simulink model "model"  (R2019a)
settings: Solver=VariableStepAuto  StartTime=0.0  StopTime=Tf  RelTol=5e-3
values from neighbouring files (symbols this model uses):
  d = 0.01    [RUN_model.m]    (also in testing.m; training.m)
  f = 10    [RUN_model.m]    (also in testing.m; training.m)
  J = 0.01    [RUN_model.m]    (also in testing.m; training.m)
  Kb = 0.0301    [RUN_model.m]    (also in testing.m; training.m)
  Kt = 0.03    [RUN_model.m]    (also in testing.m; training.m)
  L = 20e-2    (= 0.2)    [RUN_model.m]    (also in testing.m; training.m)
  La = 0.94e-3    (= 0.00094)    [RUN_model.m]    (also in testing.m; training.m)
  M = 1000e-3    (= 1)    [RUN_model.m]    (also in testing.m; training.m)
  mode = 1    [testing.m]    (also in training.m)
  N = 10    [RUN_model.m]    (also in testing.m; training.m)
  R = 0.02    [RUN_model.m]    (also in testing.m; training.m)
  Ra = 1    [RUN_model.m]    (also in testing.m; training.m)
  robot_path = [x;y]    [path_generator.m]    (also in training.m = [0;0])
  tau_b = 1    [RUN_model.m]    (also in testing.m = 0; training.m = 0)
  theta_init = deg2rad(0)    [RUN_model.m]    (also in testing.m; training.m)
  vol_gain = 1    [RUN_model.m]    (also in testing.m = 10; training.m = 10)
  xa_init = 0    [RUN_model.m]    (also in testing.m; training.m)
  ya_init = 0    [RUN_model.m]    (also in testing.m; training.m)
libraries: simulink x11, fuzblock x2, rllib x1
settings Model: Creator=omank  LastModifiedBy=omank

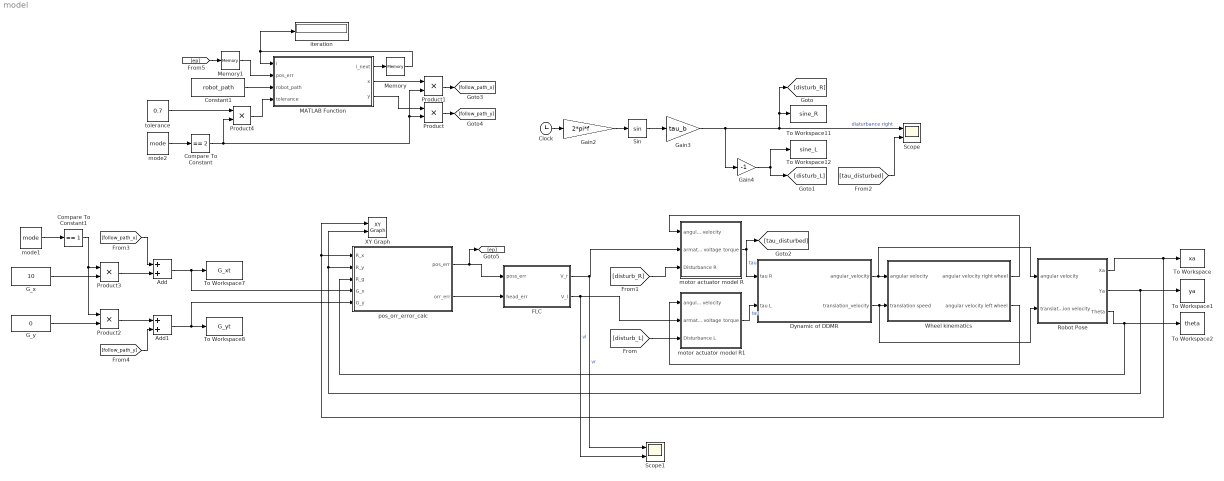
== system model ==
  Add : Sum
  Add1 : Sum
  Clock : Clock
  Compare To Constant : simulink/Logic and Bit Operations/Compare To Constant  relop===  const=2  OutDataTypeStr=boolean
  Compare To Constant1 : simulink/Logic and Bit Operations/Compare To Constant  relop===  const=1  OutDataTypeStr=boolean
  Constant1 : Constant  Value=robot_path
  Dynamic of DDMR : Subsystem
  FLC : Subsystem
  G_x : Constant  Value=10
  G_y : Constant  Value=0
  Gain2 : Gain  Gain=2*pi*f
  Gain3 : Gain  Gain=tau_b
  Gain4 : Gain  Gain=-1
  MATLAB Function : MATLAB Function  TreatAsAtomicUnit=on
  Memory : Memory  InitialCondition=1
  Memory1 : Memory  InitialCondition=1
  Product{,1..4} (5 alike) : Product
  Robot Pose : Subsystem
  Scope : Scope  NumInputPorts=2
  Scope1 : Scope  NumInputPorts=2
  Sin : Trigonometry
  To Workspace : ToWorkspace  VariableName=xa  SampleTime=-1
      settings: Save2DSignal=2-D array (concatenate along first dimension)
  To Workspace1 : ToWorkspace  VariableName=ya  SampleTime=-1
      settings: Save2DSignal=2-D array (concatenate along first dimension)
  To Workspace11 : ToWorkspace  VariableName=sine_R  SampleTime=-1
  To Workspace12 : ToWorkspace  VariableName=sine_L  SampleTime=-1
  To Workspace2 : ToWorkspace  VariableName=theta  SampleTime=-1
      settings: Save2DSignal=2-D array (concatenate along first dimension)
  To Workspace7 : ToWorkspace  VariableName=G_xt  SampleTime=-1
  To Workspace8 : ToWorkspace  VariableName=G_yt  SampleTime=-1
  Wheel kinematics : Subsystem
  XY Graph : simulink/Sinks/XY Graph  xmin=-15  xmax=15  ymin=-15  ymax=15  st=-1
  iteration : Display
  mode1 : Constant  Value=mode
  mode2 : Constant  Value=mode
  motor actuator model R : Subsystem
  motor actuator model R1 : Subsystem
  pos_orr_error_calc : MATLAB Function  TreatAsAtomicUnit=on
  tolerance : Constant  Value=0.7
  wires:
  Dynamic of DDMR/1(angular_velocity) -> Robot Pose/1(angular velocity), Wheel kinematics/1(angular velocity)
  Dynamic of DDMR/2(translation_velocity) -> Robot Pose/2(translation velocity), Wheel kinematics/2(translation speed)
  motor actuator model R/1(torque) -> [tau_disturbed], Dynamic of DDMR/1(tau R)  "tau"
  motor actuator model R1/1(torque) -> Dynamic of DDMR/2(tau L)  "tau"
  Wheel kinematics/1(angular velocity right wheel) -> motor actuator model R/1(angular velocity)
  Wheel kinematics/2(angular velocity left wheel) -> motor actuator model R1/1(angular velocity)
  Robot Pose/3(Theta) -> To Workspace2/1, pos_orr_error_calc/3(R_g)
  pos_orr_error_calc/1(pos_err) -> [ep], FLC/1(poss_err)
  Clock/1 -> Gain2/1
  Gain2/1 -> Sin/1
  Sin/1 -> Gain3/1
  Gain3/1 -> To Workspace11/1, [disturb_R], Scope/1, Gain4/1  "diaturbance right"
  Gain4/1 -> To Workspace12/1, [disturb_L]
  [disturb_R] -> motor actuator model R/3(Disturbance R)
  [disturb_L] -> motor actuator model R1/3(Disturbance L)
  [tau_disturbed] -> Scope/2
  pos_orr_error_calc/2(orr_err) -> FLC/2(head_err)
  FLC/1(V_r) -> Scope1/1, motor actuator model R/2(armature voltage)  "vr"
  FLC/2(V_l) -> Scope1/2, motor actuator model R1/2(armature voltage)  "vl"
  Add1/1 -> pos_orr_error_calc/5(G_y), To Workspace8/1
  Compare To Constant/1 -> Product4/2, Product1/2, Product/2
  Robot Pose/1(Xa) -> To Workspace/1, XY Graph/1, pos_orr_error_calc/1(R_x)
  Constant1/1 -> MATLAB Function/3(robot_path)
  Product4/1 -> MATLAB Function/4(tolerance)
  Memory/1 -> iteration/1, MATLAB Function/1(i)
  Product2/1 -> Add1/1
  G_x/1 -> Product3/2
  G_y/1 -> Product2/2
  mode1/1 -> Compare To Constant1/1
  MATLAB Function/1(i_next) -> Memory/1
  Product1/1 -> [follow_path_x]
  MATLAB Function/2(x) -> Product1/1
  Memory1/1 -> MATLAB Function/2(pos_err)
  MATLAB Function/3(y) -> Product/1
  Robot Pose/2(Ya) -> To Workspace1/1, XY Graph/2, pos_orr_error_calc/2(R_y)
  [ep] -> Memory1/1
  mode2/1 -> Compare To Constant/1
  Compare To Constant1/1 -> Product2/1, Product3/1
  Product3/1 -> Add/2
  Product/1 -> [follow_path_y]
  Add/1 -> pos_orr_error_calc/4(G_x), To Workspace7/1
  [follow_path_y] -> Add1/2
  [follow_path_x] -> Add/1
  tolerance/1 -> Product4/1

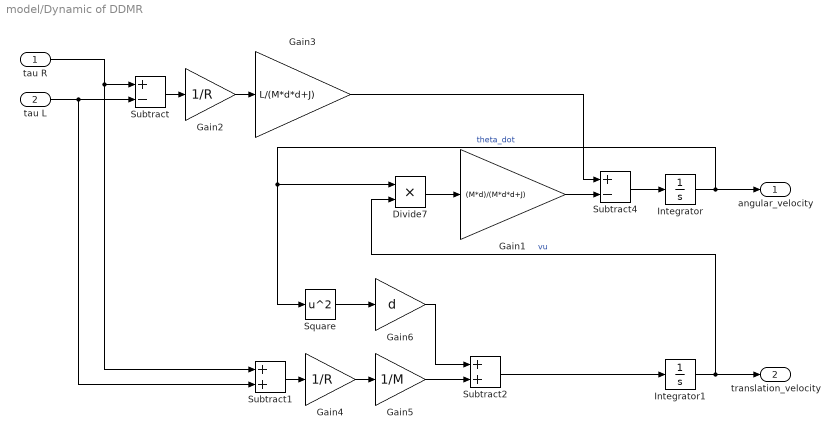
== system model/Dynamic of DDMR ==
  tau R : Inport
  tau L : Inport  Port=2
  Divide7 : Product  Inputs=**
  Gain1 : Gain  Gain=(M*d)/(M*d*d+J)
  Gain2 : Gain  Gain=1/R
  Gain3 : Gain  Gain=L/(M*d*d+J)
  Gain4 : Gain  Gain=1/R
  Gain5 : Gain  Gain=1/M
  Gain6 : Gain  Gain=d
  Integrator : Integrator
  Integrator1 : Integrator
  Square : Math  Operator=square  SaturateOnIntegerOverflow=on
  Subtract : Sum  Inputs=+-
  Subtract1 : Sum
  Subtract2 : Sum
  Subtract4 : Sum  Inputs=+-
  angular_velocity : Outport
  translation_velocity : Outport  Port=2
  wires:
  tau R/1 -> Subtract1/1, Subtract/1
  tau L/1 -> Subtract1/2, Subtract/2
  Integrator/1 -> Square/1, Divide7/1, angular_velocity/1  "theta_dot"
  Gain1/1 -> Subtract4/2
  Divide7/1 -> Gain1/1
  Integrator1/1 -> Divide7/2, translation_velocity/1  "vu"
  Gain3/1 -> Subtract4/1
  Subtract/1 -> Gain2/1
  Gain2/1 -> Gain3/1
  Subtract4/1 -> Integrator/1
  Subtract1/1 -> Gain4/1
  Gain4/1 -> Gain5/1
  Gain5/1 -> Subtract2/2
  Square/1 -> Gain6/1
  Gain6/1 -> Subtract2/1
  Subtract2/1 -> Integrator1/1

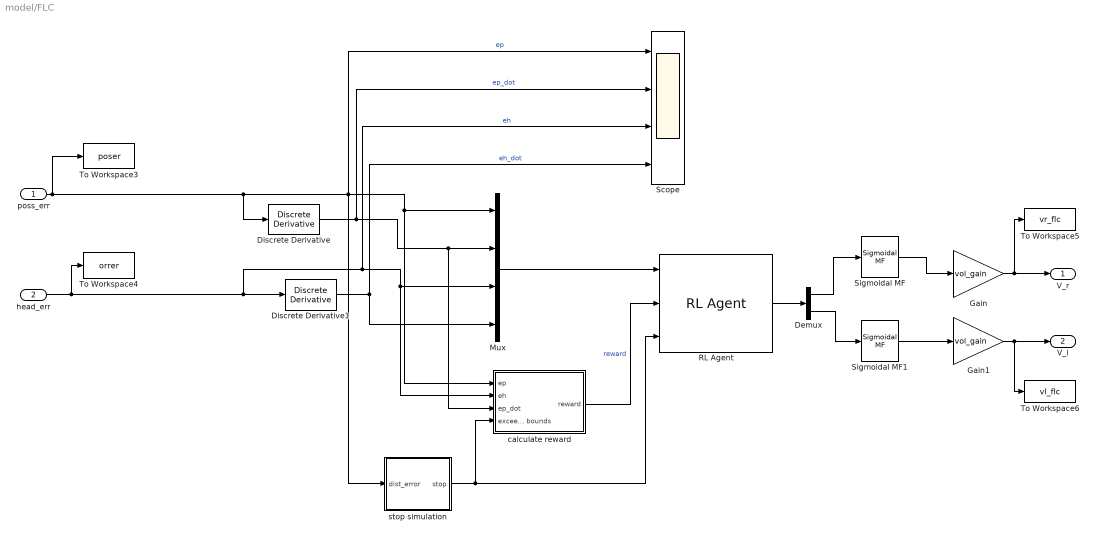
== system model/FLC ==
  poss_err : Inport
  head_err : Inport  Port=2
  Demux : Demux  Outputs=2
  Discrete Derivative : simulink/Discrete/Discrete Derivative  gainval=1.0  ICPrevScaledInput=0.0  OutMin=[]  OutMax=[]  OutDataType=fixdt(1, 16)  OutScaling=2^-10  DoSatur=off
  Discrete Derivative1 : simulink/Discrete/Discrete Derivative  gainval=1.0  ICPrevScaledInput=0.0  OutMin=[]  OutMax=[]  OutDataType=fixdt(1, 16)  OutScaling=2^-10  DoSatur=off
  Gain : Gain  Gain=vol_gain
  Gain1 : Gain  Gain=vol_gain
  Mux : Mux
  RL Agent : rllib/RL Agent  Agent=agent  ProvideReward=on  ProvideIsDone=on  ProvideCumRwd=off  TreatAsDirectFeedthrough=on  CollectLoggedSignals=on  CollectModelStates=on
      settings: SourceProductName=Reinforcement Learning Toolbox
  Scope : Scope  NumInputPorts=4
  Sigmoidal MF : fuzblock/Membership  Functions/Sigmoidal MF  a=-1  c=0
      settings: SourceProductName=Fuzzy Logic Toolbox  SourceProductBaseCode=FL
  Sigmoidal MF1 : fuzblock/Membership  Functions/Sigmoidal MF  a=-1  c=0
      settings: SourceProductName=Fuzzy Logic Toolbox  SourceProductBaseCode=FL
  To Workspace3 : ToWorkspace  VariableName=poser  SampleTime=-1
  To Workspace4 : ToWorkspace  VariableName=orrer  SampleTime=-1
  To Workspace5 : ToWorkspace  VariableName=vr_flc  SaveFormat=Structure With Time  SampleTime=-1
  To Workspace6 : ToWorkspace  VariableName=vl_flc  SaveFormat=Structure With Time  SampleTime=-1
  calculate reward : Subsystem
  stop simulation : Subsystem
  V_r : Outport
  V_l : Outport  Port=2
  wires:
  Gain/1 -> To Workspace5/1, V_r/1
  Gain1/1 -> To Workspace6/1, V_l/1
  poss_err/1 -> Discrete Derivative/1, stop simulation/1(dist_error), calculate reward/1(ep), Mux/1, Scope/1, To Workspace3/1  "ep"
  head_err/1 -> Discrete Derivative1/1, calculate reward/2(eh), Mux/3, Scope/3, To Workspace4/1  "eh"
  RL Agent/1 -> Demux/1
  calculate reward/1(reward) -> RL Agent/2  "reward"
  stop simulation/1(stop) -> calculate reward/4(exceeds bounds), RL Agent/3
  Mux/1 -> RL Agent/1
  Discrete Derivative/1 -> calculate reward/3(ep_dot), Mux/2, Scope/2  "ep_dot"
  Discrete Derivative1/1 -> Mux/4, Scope/4  "eh_dot"
  Demux/1 -> Sigmoidal MF/1
  Demux/2 -> Sigmoidal MF1/1
  Sigmoidal MF/1 -> Gain/1
  Sigmoidal MF1/1 -> Gain1/1

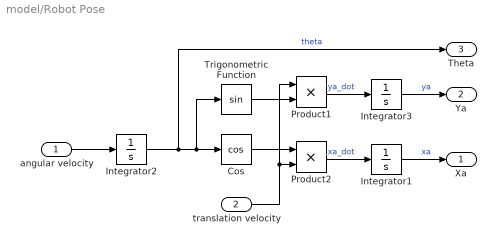
== system model/Robot Pose ==
  angular velocity : Inport
  translation velocity : Inport  Port=2
  Cos : Trigonometry  Operator=cos
  Integrator1 : Integrator  InitialCondition=xa_init
  Integrator2 : Integrator  InitialCondition=theta_init
  Integrator3 : Integrator  InitialCondition=ya_init
  Product1 : Product  Inputs=**
  Product2 : Product  Inputs=**
  Trigonometric Function : Trigonometry
  Xa : Outport
  Ya : Outport  Port=2
  Theta : Outport  Port=3
  wires:
  Trigonometric Function/1 -> Product1/2
  Integrator3/1 -> Ya/1  "ya"
  Product1/1 -> Integrator3/1  "ya_dot"
  Integrator1/1 -> Xa/1  "xa"
  Product2/1 -> Integrator1/1  "xa_dot"
  angular velocity/1 -> Integrator2/1
  Integrator2/1 -> Theta/1, Trigonometric Function/1, Cos/1  "theta"
  Cos/1 -> Product2/1
  translation velocity/1 -> Product2/2, Product1/1

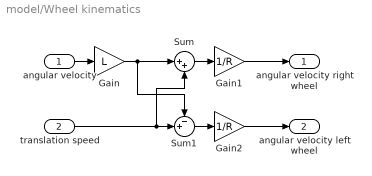
== system model/Wheel kinematics ==
  angular velocity : Inport
  translation speed : Inport  Port=2
  Gain : Gain  Gain=L
  Gain1 : Gain  Gain=1/R
  Gain2 : Gain  Gain=1/R
  Sum : Sum  Inputs=|++
  Sum1 : Sum  Inputs=-+|
  angular velocity right wheel : Outport
  angular velocity left wheel : Outport  Port=2
  wires:
  translation speed/1 -> Sum/2, Sum1/2
  angular velocity/1 -> Gain/1
  Gain/1 -> Sum1/1, Sum/1
  Sum/1 -> Gain1/1
  Gain1/1 -> angular velocity right wheel/1
  Sum1/1 -> Gain2/1
  Gain2/1 -> angular velocity left wheel/1

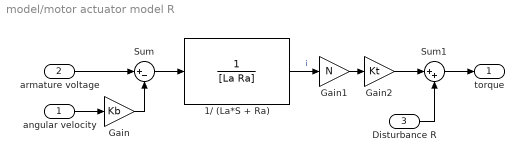
== system model/motor actuator model R ==
  angular velocity : Inport
  armature voltage : Inport  Port=2
  Disturbance R : Inport  Port=3
  1/ (La*S + Ra) : TransferFcn  Denominator=[La Ra]
  Gain : Gain  Gain=Kb
  Gain1 : Gain  Gain=N
  Gain2 : Gain  Gain=Kt
  Sum : Sum  Inputs=|+-
  Sum1 : Sum  Inputs=|++
  torque : Outport
  wires:
  armature voltage/1 -> Sum/1
  Sum/1 -> 1/ (La*S + Ra)/1
  angular velocity/1 -> Gain/1
  Gain/1 -> Sum/2
  1/ (La*S + Ra)/1 -> Gain1/1  "i"
  Gain1/1 -> Gain2/1
  Sum1/1 -> torque/1
  Gain2/1 -> Sum1/1
  Disturbance R/1 -> Sum1/2

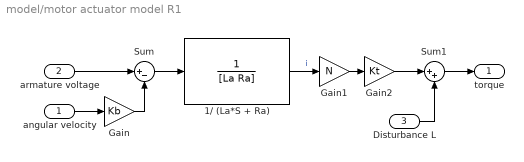
== system model/motor actuator model R1 ==
  angular velocity : Inport
  armature voltage : Inport  Port=2
  Disturbance L : Inport  Port=3
  1/ (La*S + Ra) : TransferFcn  Denominator=[La Ra]
  Gain : Gain  Gain=Kb
  Gain1 : Gain  Gain=N
  Gain2 : Gain  Gain=Kt
  Sum : Sum  Inputs=|+-
  Sum1 : Sum  Inputs=|++
  torque : Outport
  wires:
  armature voltage/1 -> Sum/1
  Sum/1 -> 1/ (La*S + Ra)/1
  angular velocity/1 -> Gain/1
  Gain/1 -> Sum/2
  1/ (La*S + Ra)/1 -> Gain1/1  "i"
  Gain1/1 -> Gain2/1
  Sum1/1 -> torque/1
  Disturbance L/1 -> Sum1/2
  Gain2/1 -> Sum1/1

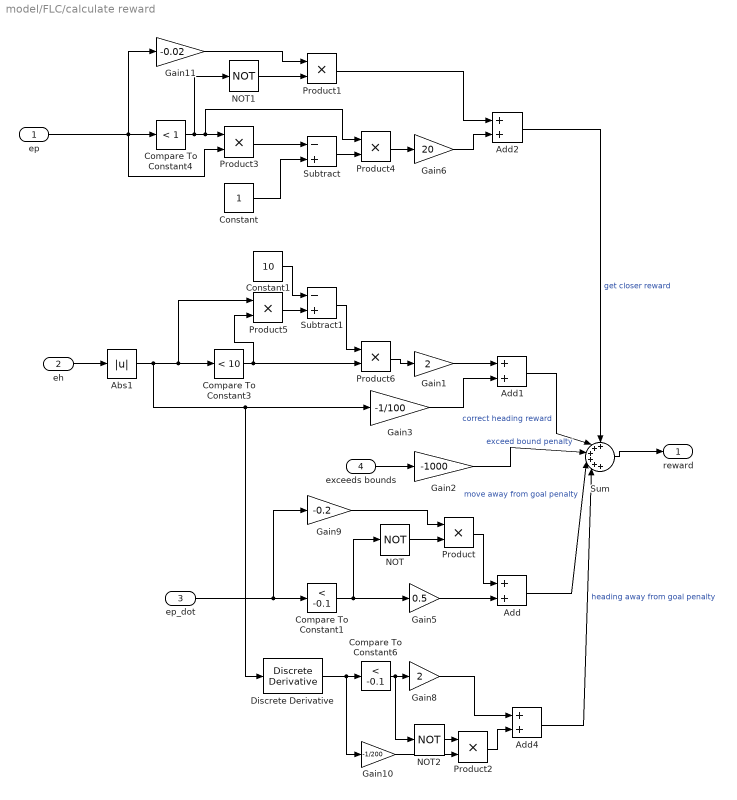
== system model/FLC/calculate reward ==
  ep : Inport
  eh : Inport  Port=2
  ep_dot : Inport  Port=3
  exceeds bounds : Inport  Port=4
  Abs1 : Abs
  Add{,1..2,4} (4 alike) : Sum
  Compare To Constant1 : simulink/Logic and Bit Operations/Compare To Constant  relop=<  const=-0.1  OutDataTypeStr=boolean
  Compare To Constant3 : simulink/Logic and Bit Operations/Compare To Constant  relop=<  const=10  OutDataTypeStr=boolean
  Compare To Constant4 : simulink/Logic and Bit Operations/Compare To Constant  relop=<  const=1  OutDataTypeStr=boolean
  Compare To Constant6 : simulink/Logic and Bit Operations/Compare To Constant  relop=<  const=-0.1  OutDataTypeStr=boolean
  Constant : Constant
  Constant1 : Constant  Value=10
  Discrete Derivative : simulink/Quick Insert/Discrete/Discrete Derivative  gainval=1.0  ICPrevScaledInput=0.0  OutMin=[]  OutMax=[]  OutDataType=fixdt(1, 16)  OutScaling=2^-10  DoSatur=off
      settings: SourceProductName=Simulink  SourceProductBaseCode=SL
  Gain1 : Gain  Gain=2
  Gain10 : Gain  Gain=-1/200
  Gain11 : Gain  Gain=-0.02
  Gain2 : Gain  Gain=-1000
  Gain3 : Gain  Gain=-1/100
  Gain5 : Gain  Gain=0.5
  Gain6 : Gain  Gain=20
  Gain8 : Gain  Gain=2
  Gain9 : Gain  Gain=-0.2
  NOT : Logic  Operator=NOT  IconShape=distinctive  AllPortsSameDT=off  OutDataTypeStr=boolean
  NOT1 : Logic  Operator=NOT  IconShape=distinctive  AllPortsSameDT=off  OutDataTypeStr=boolean
  NOT2 : Logic  Operator=NOT  IconShape=distinctive  AllPortsSameDT=off  OutDataTypeStr=boolean
  Product{,1..6} (7 alike) : Product
  Subtract : Sum  Inputs=-+
  Subtract1 : Sum  Inputs=-+
  Sum : Sum  Inputs=++++++
  reward : Outport
  wires:
  eh/1 -> Abs1/1
  Compare To Constant1/1 -> NOT/1, Gain5/1
  ep_dot/1 -> Gain9/1, Compare To Constant1/1
  NOT/1 -> Product/2
  NOT1/1 -> Product1/2
  Compare To Constant4/1 -> Product4/1, Product3/1, NOT1/1
  Product/1 -> Add/1
  Gain5/1 -> Add/2
  Gain1/1 -> Add1/1
  Gain3/1 -> Add1/2
  Product1/1 -> Add2/1
  Add1/1 -> Sum/2  "correct heading reward"
  Add2/1 -> Sum/1  "get closer reward"
  Gain2/1 -> Sum/3  "exceed bound penalty"
  Add/1 -> Sum/4  "move away from goal penalty"
  Sum/1 -> reward/1
  Constant/1 -> Subtract/2
  Gain6/1 -> Add2/2
  Gain8/1 -> Add4/1
  Discrete Derivative/1 -> Gain10/1, Compare To Constant6/1
  Abs1/1 -> Product5/1, Compare To Constant3/1, Discrete Derivative/1, Gain3/1
  Compare To Constant6/1 -> NOT2/1, Gain8/1
  NOT2/1 -> Product2/1
  Gain9/1 -> Product/1
  Gain10/1 -> Product2/2
  Product2/1 -> Add4/2
  Add4/1 -> Sum/5  "heading away from goal penalty"
  Gain11/1 -> Product1/1
  ep/1 -> Product3/2, Gain11/1, Compare To Constant4/1
  Product3/1 -> Subtract/1
  Subtract/1 -> Product4/2
  Product4/1 -> Gain6/1
  exceeds bounds/1 -> Gain2/1
  Compare To Constant3/1 -> Product5/2, Product6/2
  Product5/1 -> Subtract1/2
  Constant1/1 -> Subtract1/1
  Subtract1/1 -> Product6/1
  Product6/1 -> Gain1/1

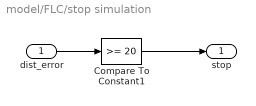
== system model/FLC/stop simulation ==
  dist_error : Inport
  Compare To Constant1 : simulink/Logic and Bit Operations/Compare To Constant  relop=>=  const=20  OutDataTypeStr=boolean
  stop : Outport
  wires:
  dist_error/1 -> Compare To Constant1/1
  Compare To Constant1/1 -> stop/1

== matlab function model/pos_orr_error_calc ==
  data: R_x input; pos_err output; orr_err output; R_y input; R_g input; G_x input; G_y input
function [pos_err,orr_err] = pos_orr_err(R_x, R_y, R_g, G_x, G_y)
    %values assignment
    rob_poss = [R_x; R_y]; %in meter
    gol_poss = [G_x; G_y]; %in meter
    gamma_r = R_g;         %in radian

    %position error
    vec_pos = gol_poss-rob_poss;
    pos_err = sqrt(sum((vec_pos).^2)); %in meter
    
    %Goal position relative to robot position to find heading error
    fTr = [cos(gamma_r) -sin(gamma_r) rob_poss(1); sin(gamma_r) cos(gamma_r) rob_poss(2); 0 0 1];
    gol_2_r_pos = (fTr)\[gol_poss(1); gol_poss(2); 1];
    %heading error
    hed_err = atan2(gol_2_r_pos(2), gol_2_r_pos(1));
    hed_err = rad2deg(hed_err);
    orr_err = hed_err; %in degree angle
end

== matlab function model/MATLAB Function ==
  data: i_next output; x output; i input; pos_err input; y output; robot_path input; tolerance input
function [i_next,x,y] = path_iterator(i, pos_err, robot_path, tolerance)
    [r,c] = size(robot_path);    
    if pos_err < tolerance
        i = i + 1;
        if i > c
            i = 1;
        end
    end
    
    x = robot_path(1,i);
    y = robot_path(2,i);
    i_next = i;
    
end
